simulink model "sampleModel20"  (R2021a)
settings: Solver=VariableStepAuto  StartTime=0.0  StopTime=10.0  RelTol=1e-3
undefined symbols (not defined in the file): DiscIntNeverNeededParam, magnitude, Newton, Raphson
libraries: simulink x274, pid_lib x17
(part 5 of 16)

== system sampleModel20/cfblk84/cfblk10/cfblk11 ==
  cfblk1 : Inport
  cfblk10 : Inport  Port=2
  cfblk11 : Inport  Port=3
  cfblk12 : Inport  Port=4
  cfblk{13..18} (6 alike) : Delay  SampleTime=1
  cfblk3 : Product  Inputs=**
  cfblk4 : Product
  cfblk5 : simulink/Math Operations/MinMax Running Resettable  Function=min  vinit=0.0
  cfblk6 : Reshape
  cfblk7 : Sqrt  Operator=rSqrt  AlgorithmType=Newton-Raphson  SaturateOnIntegerOverflow=on
  cfblk8 : Subsystem
  cfblk9 : Subsystem
  cfblk2 : Outport
  wires:
  cfblk11/1 -> cfblk5/1
  cfblk7/1 -> cfblk4/1
  cfblk3/1 -> cfblk7/1
  cfblk5/1 -> cfblk6/1
  cfblk12/1 -> cfblk9/1(cfblk1)
  cfblk8/2(cfblk7) -> cfblk9/2(cfblk6)
  cfblk1/1 -> cfblk2/1
  cfblk10/1 -> cfblk9/3(cfblk7)
  cfblk4/1 -> cfblk8/2(cfblk5)
  cfblk8/1(cfblk2) -> cfblk13/1
  cfblk13/1 -> cfblk4/2
  cfblk9/1(cfblk2) -> cfblk14/1
  cfblk14/1 -> cfblk3/2
  cfblk9/2(cfblk8) -> cfblk15/1
  cfblk15/1 -> cfblk8/1(cfblk1)
  cfblk9/3(cfblk9) -> cfblk16/1
  cfblk16/1 -> cfblk8/3(cfblk6)
  cfblk8/3(cfblk8) -> cfblk17/1
  cfblk17/1 -> cfblk3/1
  cfblk6/1 -> cfblk18/1
  cfblk18/1 -> cfblk5/2

== system sampleModel20/cfblk84/cfblk10/cfblk9 ==
  cfblk1 : Inport
  cfblk9 : Inport  Port=2
  cfblk10 : Inport  Port=3
  cfblk11 : Delay  SampleTime=1
  cfblk3 : simulink/Math Operations/Slider Gain  gain=1  low=0  high=2
  cfblk4 : Squeeze
  cfblk5 : Math  Operator=log  SaturateOnIntegerOverflow=on
  cfblk6 : PermuteDimensions
  cfblk7 : Trigonometry
  cfblk8 : Subsystem
  cfblk2 : Outport
  wires:
  cfblk9/1 -> cfblk8/1(cfblk1)
  cfblk3/1 -> cfblk6/1
  cfblk1/1 -> cfblk5/1
  cfblk8/1(cfblk2) -> cfblk7/1
  cfblk6/1 -> cfblk4/1
  cfblk5/1 -> cfblk3/1, cfblk8/5(cfblk11), cfblk8/6(cfblk12), cfblk8/7(cfblk13)
  cfblk4/1 -> cfblk8/2(cfblk8)
  cfblk10/1 -> cfblk8/4(cfblk10), cfblk2/1
  cfblk7/1 -> cfblk11/1
  cfblk11/1 -> cfblk8/3(cfblk9)

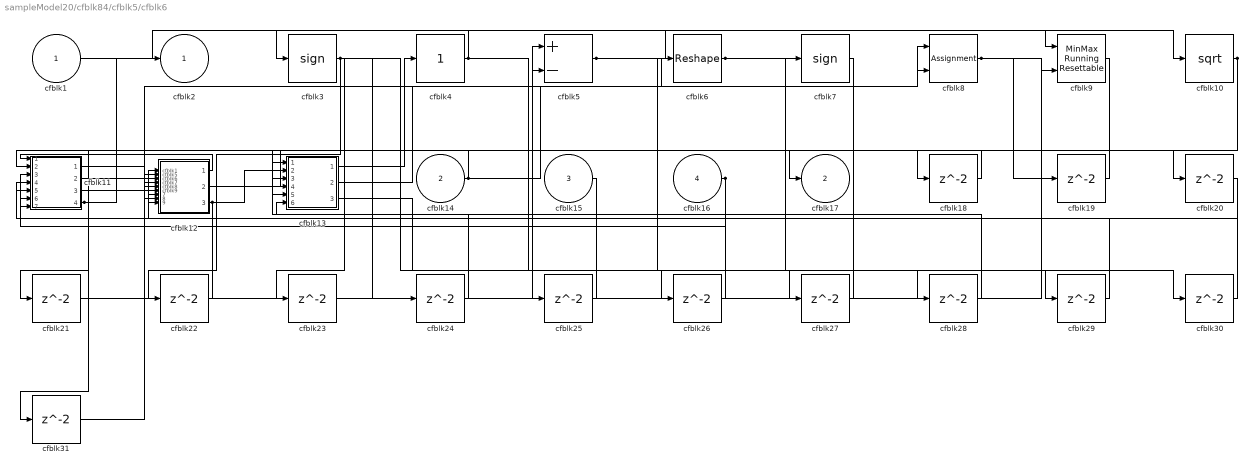
== system sampleModel20/cfblk84/cfblk5/cfblk6 ==
  cfblk1 : Inport
  cfblk14 : Inport  Port=2
  cfblk15 : Inport  Port=3
  cfblk16 : Inport  Port=4
  cfblk10 : Sqrt  SaturateOnIntegerOverflow=on
  cfblk11 : Subsystem
  cfblk12 : Subsystem
  cfblk13 : Subsystem
  cfblk{18..31} (14 alike) : Delay  SampleTime=1
  cfblk3 : Signum
  cfblk4 : simulink/Math Operations/Slider Gain  gain=1  low=0  high=2
  cfblk5 : Sum  Inputs=+-
  cfblk6 : Reshape
  cfblk7 : Signum
  cfblk8 : Assignment  DiagnosticForDimensions=Warning  IndexOptions=Index vector (dialog)  Indices=1  OutputSizes=1
  cfblk9 : simulink/Math Operations/MinMax Running Resettable  Function=min  vinit=0.0
  cfblk2 : Outport
  cfblk17 : Outport  Port=2
  wires:
  cfblk12/1(cfblk2) -> cfblk11/1(cfblk1)
  cfblk8/1 -> cfblk19/1, cfblk20/1
  cfblk15/1 -> cfblk12/1(cfblk1)
  cfblk12/2(cfblk13) -> cfblk17/1
  cfblk14/1 -> cfblk12/2(cfblk5), cfblk8/2
  cfblk16/1 -> cfblk11/3(cfblk7), cfblk12/7(cfblk10)
  cfblk13/1(cfblk2) -> cfblk4/1
  cfblk4/1 -> cfblk3/1, cfblk26/1
  cfblk5/1 -> cfblk10/1, cfblk30/1
  cfblk1/1 -> cfblk9/1
  cfblk13/2(cfblk15) -> cfblk6/1
  cfblk6/1 -> cfblk7/1, cfblk28/1
  cfblk3/1 -> cfblk22/1, cfblk23/1, cfblk24/1, cfblk25/1
  cfblk11/2(cfblk12) -> cfblk8/1
  cfblk10/1 -> cfblk13/5(cfblk13), cfblk21/1
  cfblk9/1 -> cfblk12/5(cfblk8)
  cfblk11/3(cfblk13) -> cfblk5/1
  cfblk11/4(cfblk14) -> cfblk2/1, cfblk31/1
  cfblk12/3(cfblk14) -> cfblk11/6(cfblk10), cfblk13/2(cfblk10), cfblk13/4(cfblk12)
  cfblk11/1(cfblk2) -> cfblk18/1
  cfblk18/1 -> cfblk12/4(cfblk7)
  cfblk19/1 -> cfblk11/2(cfblk6)
  cfblk20/1 -> cfblk11/7(cfblk11)
  cfblk21/1 -> cfblk9/2
  cfblk22/1 -> cfblk11/5(cfblk9)
  cfblk23/1 -> cfblk5/2
  cfblk24/1 -> cfblk13/3(cfblk11)
  cfblk25/1 -> cfblk13/6(cfblk14)
  cfblk26/1 -> cfblk12/9(cfblk12)
  cfblk7/1 -> cfblk27/1
  cfblk27/1 -> cfblk11/4(cfblk8)
  cfblk28/1 -> cfblk13/1(cfblk1)
  cfblk13/3(cfblk16) -> cfblk29/1
  cfblk29/1 -> cfblk12/3(cfblk6)
  cfblk30/1 -> cfblk12/8(cfblk11)
  cfblk31/1 -> cfblk12/6(cfblk9)

== system sampleModel20/cfblk84/cfblk5/cfblk7 ==
  cfblk1 : Inport
  cfblk9 : Inport  Port=2
  cfblk10 : Inport  Port=3
  cfblk{11..15} (5 alike) : Delay  SampleTime=1
  cfblk3 : Product  Inputs=*
  cfblk4 : Signum
  cfblk5 : Subsystem
  cfblk6 : Subsystem
  cfblk7 : Subsystem
  cfblk8 : Subsystem
  cfblk2 : Outport
  wires:
  cfblk9/1 -> cfblk8/1(cfblk1), cfblk8/7(cfblk11), cfblk6/4(cfblk10)
  cfblk4/1 -> cfblk6/1(cfblk1), cfblk5/3(cfblk12), cfblk8/6(cfblk10), cfblk5/6(cfblk15)
  cfblk3/1 -> cfblk6/2(cfblk8), cfblk7/4(cfblk12)
  cfblk1/1 -> cfblk4/1, cfblk7/3(cfblk11)
  cfblk10/1 -> cfblk3/1, cfblk7/5(cfblk13), cfblk5/5(cfblk14)
  cfblk5/1(cfblk2) -> cfblk2/1
  cfblk5/2(cfblk17) -> cfblk8/3(cfblk7), cfblk8/5(cfblk9), cfblk7/6(cfblk14)
  cfblk6/1(cfblk2) -> cfblk5/1(cfblk1), cfblk5/7(cfblk16)
  cfblk8/1(cfblk2) -> cfblk7/1(cfblk1)
  cfblk8/2(cfblk12) -> cfblk7/2(cfblk10), cfblk14/1, cfblk15/1
  cfblk7/1(cfblk2) -> cfblk11/1
  cfblk11/1 -> cfblk8/2(cfblk6)
  cfblk7/2(cfblk15) -> cfblk12/1
  cfblk12/1 -> cfblk6/3(cfblk9)
  cfblk7/3(cfblk16) -> cfblk13/1
  cfblk13/1 -> cfblk8/4(cfblk8)
  cfblk14/1 -> cfblk5/2(cfblk11)
  cfblk15/1 -> cfblk5/4(cfblk13)

== system sampleModel20/cfblk84/cfblk5/cfblk8 ==
  cfblk1 : Inport
  cfblk9 : Inport  Port=2
  cfblk10 : Inport  Port=3
  cfblk11 : Inport  Port=4
  cfblk12 : Inport  Port=5
  cfblk14 : Delay  SampleTime=1
  cfblk15 : Delay  SampleTime=1
  cfblk16 : Delay  SampleTime=1
  cfblk3 : ComplexToRealImag
  cfblk4 : Squeeze
  cfblk5 : simulink/Math Operations/Slider Gain  gain=1  low=0  high=2
  cfblk6 : Assignment  DiagnosticForDimensions=Warning  IndexOptions=Index vector (dialog)  Indices=1  OutputSizes=1
  cfblk7 : Subsystem
  cfblk8 : Subsystem
  cfblk2 : Outport
  cfblk13 : Outport  Port=2
  wires:
  cfblk12/1 -> cfblk13/1
  cfblk9/1 -> cfblk8/1(cfblk1)
  cfblk11/1 -> cfblk8/2(cfblk5), cfblk7/6(cfblk13), cfblk8/5(cfblk8)
  cfblk7/1(cfblk2) -> cfblk5/1
  cfblk5/1 -> cfblk4/1
  cfblk10/1 -> cfblk7/1(cfblk1)
  cfblk8/1(cfblk2) -> cfblk2/1
  cfblk3/1 -> cfblk7/3(cfblk10)
  cfblk8/2(cfblk9) -> cfblk3/1
  cfblk1/1 -> cfblk8/3(cfblk6)
  cfblk7/2(cfblk14) -> cfblk6/1
  cfblk3/2 -> cfblk7/4(cfblk11)
  cfblk7/3(cfblk15) -> cfblk6/2, cfblk16/1
  cfblk4/1 -> cfblk14/1
  cfblk14/1 -> cfblk7/2(cfblk9)
  cfblk6/1 -> cfblk15/1
  cfblk15/1 -> cfblk7/5(cfblk12)
  cfblk16/1 -> cfblk8/4(cfblk7)

== system sampleModel20/cfblk84/cfblk5/cfblk9 ==
  cfblk1 : Inport
  cfblk8 : Inport  Port=2
  cfblk9 : Inport  Port=3
  cfblk12 : Delay  SampleTime=1
  cfblk3 : Polyval  Coefs=[ +2.081618890e-019, -1.441693666e-014, +4.719686976e-010, -8.536869453e-006, +1.621573104e-001, -8.087801117e+001 ]
  cfblk4 : Product
  cfblk5 : UnaryMinus
  cfblk6 : Subsystem
  cfblk7 : Subsystem
  cfblk2 : Outport
  cfblk10 : Outport  Port=2
  cfblk11 : Outport  Port=3
  wires:
  cfblk5/1 -> cfblk10/1, cfblk7/3(cfblk6)
  cfblk3/1 -> cfblk4/1
  cfblk6/1(cfblk2) -> cfblk5/1
  cfblk9/1 -> cfblk4/2
  cfblk1/1 -> cfblk6/1(cfblk1)
  cfblk6/2(cfblk7) -> cfblk2/1
  cfblk8/1 -> cfblk6/3(cfblk6), cfblk7/2(cfblk5), cfblk7/4(cfblk7)
  cfblk7/1(cfblk2) -> cfblk3/1
  cfblk6/3(cfblk8) -> cfblk7/1(cfblk1)
  cfblk7/2(cfblk8) -> cfblk11/1
  cfblk4/1 -> cfblk12/1
  cfblk12/1 -> cfblk6/2(cfblk5)

== system sampleModel20/cfblk84/cfblk6/cfblk4 ==
  cfblk1 : Inport
  cfblk6 : Inport  Port=2
  cfblk7 : Inport  Port=3
  cfblk3 : ComplexToRealImag
  cfblk4 : Gain  Gain=[670276917.632316]
  cfblk5 : Subsystem
  cfblk2 : Outport
  wires:
  cfblk4/1 -> cfblk5/1(cfblk1)
  cfblk3/1 -> cfblk4/1
  cfblk6/1 -> cfblk5/2(cfblk8)
  cfblk1/1 -> cfblk5/3(cfblk9)
  cfblk5/1(cfblk2) -> cfblk2/1
  cfblk7/1 -> cfblk3/1
  cfblk3/2 -> cfblk5/4(cfblk10)

== system sampleModel20/cfblk84/cfblk6/cfblk5 ==
  cfblk1 : Inport
  cfblk11 : Inport  Port=2
  cfblk12 : Inport  Port=3
  cfblk13 : Inport  Port=4
  cfblk10 : Subsystem
  cfblk{14..20} (7 alike) : Delay  SampleTime=1
  cfblk3 : Signum
  cfblk4 : Sqrt  Operator=rSqrt  AlgorithmType=Newton-Raphson  SaturateOnIntegerOverflow=on
  cfblk5 : Signum
  cfblk6 : Subsystem
  cfblk7 : Subsystem
  cfblk8 : Subsystem
  cfblk9 : Subsystem
  cfblk2 : Outport
  wires:
  cfblk5/1 -> cfblk18/1, cfblk19/1, cfblk20/1
  cfblk1/1 -> cfblk4/1, cfblk8/4(cfblk8)
  cfblk10/1(cfblk2) -> cfblk7/1(cfblk1)
  cfblk11/1 -> cfblk10/2(cfblk11)
  cfblk12/1 -> cfblk6/1(cfblk1), cfblk9/4(cfblk12)
  cfblk13/1 -> cfblk3/1, cfblk9/5(cfblk13), cfblk9/6(cfblk14)
  cfblk6/1(cfblk2) -> cfblk9/1(cfblk1)
  cfblk4/1 -> cfblk10/4(cfblk13)
  cfblk10/2(cfblk15) -> cfblk9/2(cfblk10)
  cfblk3/1 -> cfblk2/1, cfblk9/3(cfblk11)
  cfblk8/2(cfblk10) -> cfblk5/1
  cfblk10/3(cfblk16) -> cfblk8/1(cfblk1)
  cfblk7/2(cfblk8) -> cfblk6/2(cfblk10)
  cfblk6/2(cfblk12) -> cfblk8/2(cfblk6), cfblk8/3(cfblk7)
  cfblk7/1(cfblk2) -> cfblk14/1
  cfblk14/1 -> cfblk10/5(cfblk14)
  cfblk9/1(cfblk2) -> cfblk15/1
  cfblk15/1 -> cfblk7/2(cfblk6)
  cfblk9/2(cfblk15) -> cfblk16/1
  cfblk16/1 -> cfblk7/3(cfblk7)
  cfblk8/1(cfblk2) -> cfblk17/1
  cfblk17/1 -> cfblk10/3(cfblk12)
  cfblk18/1 -> cfblk10/1(cfblk1)
  cfblk19/1 -> cfblk6/3(cfblk11)
  cfblk20/1 -> cfblk8/5(cfblk9)

== system sampleModel20/cfblk84/cfblk6/cfblk6 ==
  cfblk1 : Inport
  cfblk7 : Inport  Port=2
  cfblk8 : Inport  Port=3
  cfblk9 : Inport  Port=4
  cfblk10 : Inport  Port=5
  cfblk11 : Inport  Port=6
  cfblk12 : Inport  Port=7
  cfblk13 : Inport  Port=8
  cfblk14 : Inport  Port=9
  cfblk3 : Assignment  DiagnosticForDimensions=Warning  IndexOptions=Index vector (dialog)  Indices=1  OutputSizes=1
  cfblk4 : Product  Inputs=*
  cfblk5 : Subsystem
  cfblk6 : Subsystem
  cfblk2 : Outport
  cfblk15 : Outport  Port=2
  cfblk16 : Outport  Port=3
  wires:
  cfblk13/1 -> cfblk16/1, cfblk5/7(cfblk9)
  cfblk10/1 -> cfblk6/1(cfblk1)
  cfblk6/1(cfblk2) -> cfblk2/1
  cfblk8/1 -> cfblk6/2(cfblk8), cfblk5/8(cfblk10), cfblk5/10(cfblk12)
  cfblk1/1 -> cfblk3/1
  cfblk4/1 -> cfblk15/1
  cfblk5/1(cfblk2) -> cfblk4/1
  cfblk9/1 -> cfblk3/2
  cfblk6/2(cfblk9) -> cfblk5/1(cfblk1)
  cfblk12/1 -> cfblk5/2(cfblk4), cfblk5/9(cfblk11)
  cfblk11/1 -> cfblk5/3(cfblk5)
  cfblk7/1 -> cfblk5/4(cfblk6)
  cfblk14/1 -> cfblk5/5(cfblk7)
  cfblk3/1 -> cfblk5/6(cfblk8)

== system sampleModel20/cfblk84/cfblk7/cfblk10 ==
  cfblk1 : Inport
  cfblk10 : Inport  Port=2
  cfblk11 : Inport  Port=3
  cfblk12 : Inport  Port=4
  cfblk13 : Inport  Port=5
  cfblk14 : Inport  Port=6
  cfblk{18..21} (4 alike) : Delay  SampleTime=1
  cfblk3 : Product
  cfblk4 : ComplexToRealImag
  cfblk5 : ComplexToMagnitudeAngle
  cfblk6 : Subsystem
  cfblk7 : Subsystem
  cfblk8 : Subsystem
  cfblk9 : Subsystem
  cfblk2 : Outport
  cfblk15 : Outport  Port=2
  cfblk16 : Outport  Port=3
  cfblk17 : Outport  Port=4
  wires:
  cfblk4/1 -> cfblk9/1(cfblk1)
  cfblk8/1(cfblk2) -> cfblk16/1
  cfblk7/1(cfblk2) -> cfblk17/1
  cfblk10/1 -> cfblk7/1(cfblk1)
  cfblk6/1(cfblk2) -> cfblk4/1
  cfblk3/1 -> cfblk6/2(cfblk6), cfblk19/1, cfblk21/1
  cfblk9/1(cfblk2) -> cfblk7/2(cfblk7)
  cfblk5/1 -> cfblk15/1
  cfblk14/1 -> cfblk3/1
  cfblk5/2 -> cfblk3/2, cfblk6/3(cfblk7)
  cfblk4/2 -> cfblk7/3(cfblk8), cfblk20/1
  cfblk6/2(cfblk9) -> cfblk9/2(cfblk5)
  cfblk1/1 -> cfblk8/2(cfblk8), cfblk8/5(cfblk11)
  cfblk13/1 -> cfblk9/3(cfblk6)
  cfblk7/2(cfblk10) -> cfblk2/1, cfblk18/1
  cfblk8/2(cfblk14) -> cfblk7/4(cfblk9)
  cfblk6/3(cfblk10) -> cfblk9/4(cfblk7)
  cfblk12/1 -> cfblk8/3(cfblk9), cfblk9/6(cfblk9)
  cfblk8/3(cfblk15) -> cfblk5/1
  cfblk8/4(cfblk16) -> cfblk9/5(cfblk8)
  cfblk11/1 -> cfblk6/1(cfblk1), cfblk6/4(cfblk8)
  cfblk18/1 -> cfblk8/7(cfblk13)
  cfblk19/1 -> cfblk8/1(cfblk1)
  cfblk20/1 -> cfblk8/4(cfblk10)
  cfblk21/1 -> cfblk8/6(cfblk12)

== system sampleModel20/cfblk84/cfblk7/cfblk9 ==
  cfblk1 : Inport
  cfblk8 : Inport  Port=2
  cfblk9 : Inport  Port=3
  cfblk10 : Inport  Port=4
  cfblk11 : Inport  Port=5
  cfblk12 : Inport  Port=6
  cfblk15 : Delay  SampleTime=1
  cfblk3 : Sum  Inputs=|++
  cfblk4 : Product  Inputs=**
  cfblk5 : Sum  Inputs=+
  cfblk6 : Sum  Inputs=+
  cfblk7 : Subsystem
  cfblk2 : Outport
  cfblk13 : Outport  Port=2
  cfblk14 : Outport  Port=3
  wires:
  cfblk11/1 -> cfblk14/1
  cfblk7/1(cfblk2) -> cfblk5/1
  cfblk3/1 -> cfblk13/1
  cfblk9/1 -> cfblk7/1(cfblk1)
  cfblk4/1 -> cfblk3/1
  cfblk6/1 -> cfblk3/2
  cfblk12/1 -> cfblk6/1
  cfblk5/1 -> cfblk4/1, cfblk15/1
  cfblk8/1 -> cfblk7/2(cfblk12)
  cfblk7/2(cfblk16) -> cfblk2/1
  cfblk1/1 -> cfblk7/3(cfblk13)
  cfblk10/1 -> cfblk7/4(cfblk14)
  cfblk7/3(cfblk17) -> cfblk4/2
  cfblk15/1 -> cfblk7/5(cfblk15)

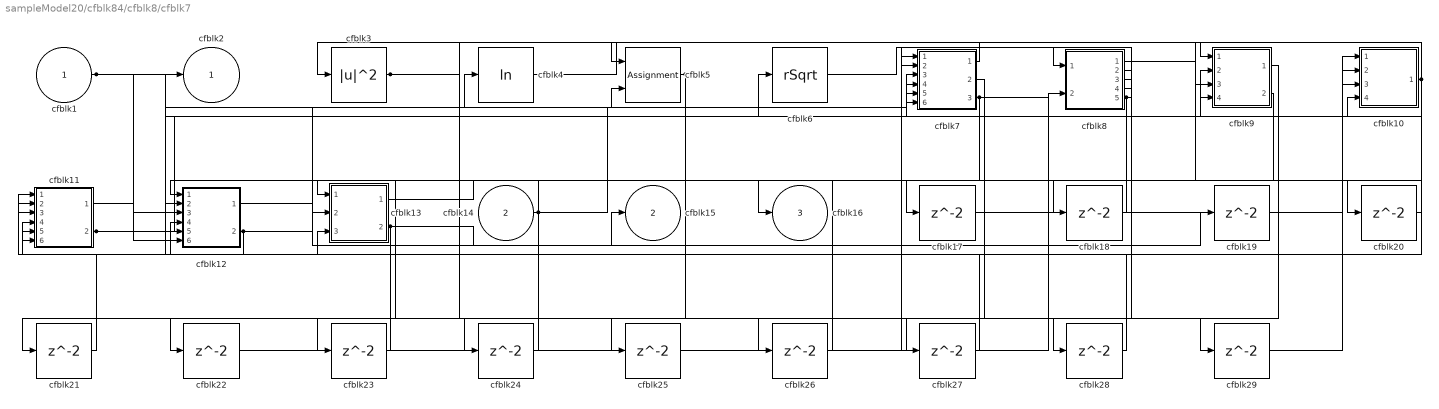
== system sampleModel20/cfblk84/cfblk8/cfblk7 ==
  cfblk1 : Inport
  cfblk14 : Inport  Port=2
  cfblk10 : Subsystem
  cfblk11 : Subsystem
  cfblk12 : Subsystem
  cfblk13 : Subsystem
  cfblk{17..29} (13 alike) : Delay  SampleTime=1
  cfblk3 : Math  Operator=magnitude^2  SaturateOnIntegerOverflow=on
  cfblk4 : Math  Operator=log  SaturateOnIntegerOverflow=on
  cfblk5 : Assignment  DiagnosticForDimensions=Warning  IndexOptions=Index vector (dialog)  Indices=1  OutputSizes=1
  cfblk6 : Sqrt  Operator=rSqrt  AlgorithmType=Newton-Raphson  SaturateOnIntegerOverflow=on
  cfblk7 : Subsystem
  cfblk8 : Subsystem
  cfblk9 : Subsystem
  cfblk2 : Outport
  cfblk15 : Outport  Port=2
  cfblk16 : Outport  Port=3
  wires:
  cfblk4/1 -> cfblk9/1(cfblk1)
  cfblk5/1 -> cfblk4/1, cfblk24/1
  cfblk3/1 -> cfblk9/3(cfblk9), cfblk29/1
  cfblk11/1(cfblk2) -> cfblk2/1
  cfblk6/1 -> cfblk8/1(cfblk1)
  cfblk11/2(cfblk15) -> cfblk6/1, cfblk5/2
  cfblk10/1(cfblk2) -> cfblk13/3(cfblk9), cfblk3/1, cfblk7/6(cfblk13)
  cfblk12/2(cfblk12) -> cfblk11/5(cfblk13), cfblk7/5(cfblk12), cfblk19/1
  cfblk1/1 -> cfblk10/4(cfblk9), cfblk12/3(cfblk8), cfblk12/6(cfblk11)
  cfblk13/2(cfblk10) -> cfblk15/1, cfblk12/4(cfblk9)
  cfblk14/1 -> cfblk12/1(cfblk1), cfblk7/4(cfblk11), cfblk11/4(cfblk12)
  cfblk8/3(cfblk14) -> cfblk7/2(cfblk9)
  cfblk7/1(cfblk2) -> cfblk5/1
  cfblk8/4(cfblk15) -> cfblk7/3(cfblk10)
  cfblk7/3(cfblk15) -> cfblk9/2(cfblk8), cfblk9/4(cfblk10), cfblk16/1
  cfblk8/5(cfblk16) -> cfblk26/1, cfblk27/1, cfblk28/1
  cfblk13/1(cfblk2) -> cfblk17/1
  cfblk17/1 -> cfblk10/2(cfblk7)
  cfblk12/1(cfblk2) -> cfblk18/1
  cfblk18/1 -> cfblk13/2(cfblk8)
  cfblk19/1 -> cfblk10/3(cfblk8)
  cfblk8/1(cfblk2) -> cfblk20/1
  cfblk20/1 -> cfblk13/1(cfblk1)
  cfblk8/2(cfblk13) -> cfblk21/1
  cfblk21/1 -> cfblk11/2(cfblk10)
  cfblk9/1(cfblk2) -> cfblk22/1
  cfblk22/1 -> cfblk7/1(cfblk1)
  cfblk9/2(cfblk11) -> cfblk23/1
  cfblk23/1 -> cfblk11/1(cfblk1)
  cfblk24/1 -> cfblk12/5(cfblk10)
  cfblk7/2(cfblk14) -> cfblk25/1
  cfblk25/1 -> cfblk8/2(cfblk12)
  cfblk26/1 -> cfblk11/3(cfblk11)
  cfblk27/1 -> cfblk11/6(cfblk14)
  cfblk28/1 -> cfblk12/2(cfblk7)
  cfblk29/1 -> cfblk10/1(cfblk1)

== system sampleModel20/cfblk84/cfblk8/cfblk8 ==
  cfblk1 : Inport
  cfblk11 : Inport  Port=2
  cfblk10 : Subsystem
  cfblk{12..16} (5 alike) : Delay  SampleTime=1
  cfblk3 : Sqrt  SaturateOnIntegerOverflow=on
  cfblk4 : Sqrt  SaturateOnIntegerOverflow=on
  cfblk5 : Signum
  cfblk6 : Polyval  Coefs=[ +2.081618890e-019, -1.441693666e-014, +4.719686976e-010, -8.536869453e-006, +1.621573104e-001, -8.087801117e+001 ]
  cfblk7 : Subsystem
  cfblk8 : Subsystem
  cfblk9 : Subsystem
  cfblk2 : Outport
  wires:
  cfblk9/1(cfblk2) -> cfblk3/1, cfblk15/1
  cfblk8/1(cfblk2) -> cfblk4/1
  cfblk1/1 -> cfblk6/1, cfblk8/2(cfblk3), cfblk7/4(cfblk12)
  cfblk6/1 -> cfblk10/2(cfblk7), cfblk2/1, cfblk8/3(cfblk4)
  cfblk7/3(cfblk16) -> cfblk5/1
  cfblk4/1 -> cfblk7/6(cfblk14), cfblk16/1
  cfblk11/1 -> cfblk9/2(cfblk7), cfblk8/4(cfblk5)
  cfblk3/1 -> cfblk7/2(cfblk10)
  cfblk8/2(cfblk6) -> cfblk10/3(cfblk8)
  cfblk10/1(cfblk2) -> cfblk9/3(cfblk8), cfblk7/3(cfblk11), cfblk7/5(cfblk13)
  cfblk8/3(cfblk7) -> cfblk10/4(cfblk9)
  cfblk7/1(cfblk2) -> cfblk12/1
  cfblk12/1 -> cfblk9/1(cfblk1)
  cfblk7/2(cfblk15) -> cfblk13/1
  cfblk13/1 -> cfblk10/1(cfblk1)
  cfblk5/1 -> cfblk14/1
  cfblk14/1 -> cfblk7/1(cfblk1)
  cfblk15/1 -> cfblk10/5(cfblk10)
  cfblk16/1 -> cfblk8/1(cfblk1)

== system sampleModel20/cfblk84/cfblk8/cfblk9 ==
  cfblk1 : Inport
  cfblk7 : Inport  Port=2
  cfblk8 : Inport  Port=3
  cfblk9 : Inport  Port=4
  cfblk11 : Delay  SampleTime=1
  cfblk12 : Delay  SampleTime=1
  cfblk13 : Delay  SampleTime=1
  cfblk3 : DiscreteStateSpace
  cfblk4 : Subsystem
  cfblk5 : Subsystem
  cfblk6 : Subsystem
  cfblk2 : Outport
  cfblk10 : Outport  Port=2
  wires:
  cfblk5/2(cfblk10) -> cfblk2/1
  cfblk5/3(cfblk11) -> cfblk3/1, cfblk6/7(cfblk16)
  cfblk7/1 -> cfblk5/1(cfblk1), cfblk6/5(cfblk14), cfblk6/6(cfblk15)
  cfblk4/1(cfblk2) -> cfblk5/2(cfblk7)
  cfblk8/1 -> cfblk5/3(cfblk8), cfblk6/2(cfblk11), cfblk6/3(cfblk12)
  cfblk3/1 -> cfblk10/1, cfblk6/1(cfblk1), cfblk6/4(cfblk13)
  cfblk9/1 -> cfblk5/4(cfblk9)
  cfblk1/1 -> cfblk4/2(cfblk5)
  cfblk5/1(cfblk2) -> cfblk11/1
  cfblk11/1 -> cfblk4/1(cfblk1)
  cfblk6/1(cfblk2) -> cfblk12/1
  cfblk12/1 -> cfblk4/3(cfblk6)
  cfblk6/2(cfblk17) -> cfblk13/1
  cfblk13/1 -> cfblk4/4(cfblk7)

== system sampleModel20/cfblk84/cfblk9/cfblk5 ==
  cfblk1 : Inport
  cfblk9 : Inport  Port=2
  cfblk10 : Inport  Port=3
  cfblk11 : Inport  Port=4
  cfblk12 : Delay  SampleTime=1
  cfblk13 : Delay  SampleTime=1
  cfblk3 : DotProduct  InputSameDT=on  OutDataTypeStr=Inherit: Inherit via internal rule
  cfblk4 : Math  Operator=log10  SaturateOnIntegerOverflow=on
  cfblk5 : simulink/Math Operations/MinMax Running Resettable  Function=min  vinit=0.0
  cfblk6 : simulink/Math Operations/Slider Gain  gain=1  low=0  high=2
  cfblk7 : Assignment  DiagnosticForDimensions=Warning  IndexOptions=Index vector (dialog)  Indices=1  OutputSizes=1
  cfblk8 : Subsystem
  cfblk2 : Outport
  wires:
  cfblk11/1 -> cfblk2/1
  cfblk5/1 -> cfblk8/1(cfblk1)
  cfblk1/1 -> cfblk7/1
  cfblk10/1 -> cfblk7/2
  cfblk3/1 -> cfblk5/1
  cfblk9/1 -> cfblk3/1
  cfblk4/1 -> cfblk6/1
  cfblk8/1(cfblk2) -> cfblk4/1
  cfblk6/1 -> cfblk12/1
  cfblk12/1 -> cfblk5/2
  cfblk8/2(cfblk8) -> cfblk13/1
  cfblk13/1 -> cfblk3/2

== system sampleModel20/cfblk84/cfblk9/cfblk6 ==
  cfblk1 : Inport
  cfblk9 : Inport  Port=2
  cfblk10 : Inport  Port=3
  cfblk11 : Inport  Port=4
  cfblk12 : Inport  Port=5
  cfblk13 : Inport  Port=6
  cfblk14 : Inport  Port=7
  cfblk15 : Inport  Port=8
  cfblk{17..21} (5 alike) : Delay  SampleTime=1
  cfblk3 : ComplexToRealImag
  cfblk4 : Subsystem
  cfblk5 : Subsystem
  cfblk6 : Subsystem
  cfblk7 : Subsystem
  cfblk8 : Subsystem
  cfblk2 : Outport
  cfblk16 : Outport  Port=2
  wires:
  cfblk8/1(cfblk2) -> cfblk16/1
  cfblk14/1 -> cfblk8/1(cfblk1), cfblk5/2(cfblk6)
  cfblk1/1 -> cfblk2/1, cfblk6/6(cfblk11)
  cfblk15/1 -> cfblk7/1(cfblk1)
  cfblk11/1 -> cfblk7/2(cfblk9), cfblk5/3(cfblk7), cfblk6/4(cfblk9)
  cfblk6/1(cfblk2) -> cfblk7/3(cfblk10), cfblk5/4(cfblk8)
  cfblk12/1 -> cfblk6/2(cfblk7), cfblk4/8(cfblk12)
  cfblk10/1 -> cfblk8/2(cfblk14), cfblk4/5(cfblk9)
  cfblk13/1 -> cfblk4/1(cfblk1), cfblk4/7(cfblk11)
  cfblk7/1(cfblk2) -> cfblk3/1
  cfblk3/2 -> cfblk4/2(cfblk6)
  cfblk8/2(cfblk15) -> cfblk7/5(cfblk12)
  cfblk9/1 -> cfblk4/3(cfblk7), cfblk6/3(cfblk8), cfblk5/5(cfblk9)
  cfblk4/2(cfblk14) -> cfblk19/1, cfblk20/1
  cfblk8/3(cfblk16) -> cfblk7/7(cfblk14), cfblk7/9(cfblk16)
  cfblk7/2(cfblk17) -> cfblk5/1(cfblk1), cfblk21/1
  cfblk5/1(cfblk2) -> cfblk4/4(cfblk8), cfblk4/6(cfblk10), cfblk4/9(cfblk13)
  cfblk3/1 -> cfblk17/1
  cfblk17/1 -> cfblk6/1(cfblk1)
  cfblk4/1(cfblk2) -> cfblk18/1
  cfblk18/1 -> cfblk7/4(cfblk11)
  cfblk19/1 -> cfblk7/6(cfblk13)
  cfblk20/1 -> cfblk7/8(cfblk15)
  cfblk21/1 -> cfblk6/5(cfblk10)

== system sampleModel20/cfblk84/cfblk9/cfblk7 ==
  cfblk1 : Inport
  cfblk9 : Inport  Port=2
  cfblk10 : Inport  Port=3
  cfblk11 : Inport  Port=4
  cfblk12 : Inport  Port=5
  cfblk{13..18} (6 alike) : Delay  SampleTime=1
  cfblk3 : Abs
  cfblk4 : simulink/Math Operations/MinMax Running Resettable  Function=min  vinit=0.0
  cfblk5 : Subsystem
  cfblk6 : Subsystem
  cfblk7 : Subsystem
  cfblk8 : Subsystem
  cfblk2 : Outport
  wires:
  cfblk10/1 -> cfblk6/1(cfblk1)
  cfblk8/1(cfblk2) -> cfblk5/1(cfblk1)
  cfblk11/1 -> cfblk2/1
  cfblk8/2(cfblk7) -> cfblk3/1
  cfblk12/1 -> cfblk7/1(cfblk1)
  cfblk1/1 -> cfblk7/3(cfblk7)
  cfblk9/1 -> cfblk5/2(cfblk5)
  cfblk7/1(cfblk2) -> cfblk8/2(cfblk6)
  cfblk5/3(cfblk8) -> cfblk6/2(cfblk6)
  cfblk5/4(cfblk9) -> cfblk6/3(cfblk7)
  cfblk7/2(cfblk11) -> cfblk4/1
  cfblk5/5(cfblk10) -> cfblk4/2
  cfblk5/1(cfblk2) -> cfblk13/1
  cfblk13/1 -> cfblk7/5(cfblk9)
  cfblk5/2(cfblk7) -> cfblk14/1
  cfblk14/1 -> cfblk7/6(cfblk10)
  cfblk6/1(cfblk2) -> cfblk15/1
  cfblk15/1 -> cfblk7/4(cfblk8)
  cfblk6/2(cfblk8) -> cfblk16/1
  cfblk16/1 -> cfblk5/3(cfblk6)
  cfblk4/1 -> cfblk17/1
  cfblk17/1 -> cfblk7/2(cfblk6)
  cfblk3/1 -> cfblk18/1
  cfblk18/1 -> cfblk8/1(cfblk1)

== system sampleModel20/cfblk85/cfblk10/cfblk6 ==
  cfblk1 : Inport
  cfblk7 : Inport  Port=2
  cfblk8 : Inport  Port=3
  cfblk9 : Inport  Port=4
  cfblk10 : Inport  Port=5
  cfblk11 : Inport  Port=6
  cfblk12 : Inport  Port=7
  cfblk14 : Delay  SampleTime=1
  cfblk3 : Subsystem
  cfblk4 : Subsystem
  cfblk5 : Subsystem
  cfblk6 : Subsystem
  cfblk2 : Outport
  cfblk13 : Outport  Port=2
  wires:
  cfblk7/1 -> cfblk6/1(cfblk1)
  cfblk12/1 -> cfblk4/1(cfblk1), cfblk3/7(cfblk15)
  cfblk10/1 -> cfblk13/1, cfblk3/4(cfblk12), cfblk3/5(cfblk13)
  cfblk11/1 -> cfblk5/1(cfblk1)
  cfblk1/1 -> cfblk4/2(cfblk11), cfblk3/3(cfblk11)
  cfblk9/1 -> cfblk4/3(cfblk12)
  cfblk8/1 -> cfblk6/2(cfblk5), cfblk3/6(cfblk14)
  cfblk6/1(cfblk2) -> cfblk5/2(cfblk10)
  cfblk3/1(cfblk2) -> cfblk6/3(cfblk6)
  cfblk3/2(cfblk16) -> cfblk6/4(cfblk7)
  cfblk4/1(cfblk2) -> cfblk2/1
  cfblk4/2(cfblk14) -> cfblk3/1(cfblk1), cfblk3/2(cfblk10)
  cfblk3/3(cfblk17) -> cfblk6/5(cfblk8)
  cfblk5/1(cfblk2) -> cfblk14/1
  cfblk14/1 -> cfblk4/4(cfblk13)

== system sampleModel20/cfblk85/cfblk9/cfblk6 ==
  cfblk1 : Inport
  cfblk6 : Inport  Port=2
  cfblk7 : Inport  Port=3
  cfblk8 : Inport  Port=4
  cfblk9 : Inport  Port=5
  cfblk3 : Gain  Gain=[-520885476.309207]
  cfblk4 : Trigonometry
  cfblk5 : Subsystem
  cfblk2 : Outport
  cfblk10 : Outport  Port=2
  wires:
  cfblk7/1 -> cfblk10/1, cfblk5/4(cfblk9)
  cfblk3/1 -> cfblk2/1
  cfblk8/1 -> cfblk5/1(cfblk1)
  cfblk6/1 -> cfblk4/1
  cfblk4/1 -> cfblk5/2(cfblk7)
  cfblk1/1 -> cfblk3/1
  cfblk9/1 -> cfblk5/3(cfblk8), cfblk5/5(cfblk10)

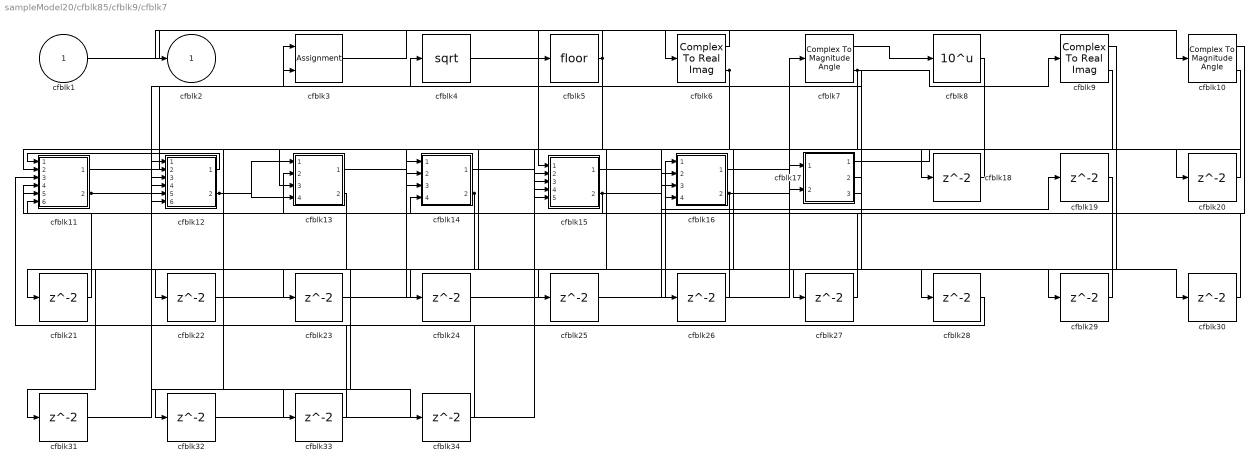
== system sampleModel20/cfblk85/cfblk9/cfblk7 ==
  cfblk1 : Inport
  cfblk10 : ComplexToMagnitudeAngle
  cfblk11 : Subsystem
  cfblk12 : Subsystem
  cfblk13 : Subsystem
  cfblk14 : Subsystem
  cfblk15 : Subsystem
  cfblk16 : Subsystem
  cfblk17 : Subsystem
  cfblk{18..34} (17 alike) : Delay  SampleTime=1
  cfblk3 : Assignment  DiagnosticForDimensions=Warning  IndexOptions=Index vector (dialog)  Indices=1  OutputSizes=1
  cfblk4 : Sqrt  SaturateOnIntegerOverflow=on
  cfblk5 : Rounding
  cfblk6 : ComplexToRealImag
  cfblk7 : ComplexToMagnitudeAngle
  cfblk8 : Math  Operator=10^u  SaturateOnIntegerOverflow=on
  cfblk9 : ComplexToRealImag
  cfblk2 : Outport
  wires:
  cfblk7/1 -> cfblk8/1
  cfblk7/2 -> cfblk9/1, cfblk25/1, cfblk26/1, cfblk27/1
  cfblk1/1 -> cfblk6/1
  cfblk11/1(cfblk2) -> cfblk4/1
  cfblk5/1 -> cfblk2/1, cfblk12/4(cfblk8)
  cfblk12/1(cfblk2) -> cfblk11/1(cfblk1)
  cfblk4/1 -> cfblk15/1(cfblk1)
  cfblk16/1(cfblk2) -> cfblk7/1
  cfblk11/2(cfblk13) -> cfblk3/1, cfblk34/1
  cfblk12/2(cfblk11) -> cfblk13/1(cfblk1), cfblk13/4(cfblk9)
  cfblk3/1 -> cfblk10/1
  cfblk14/1(cfblk2) -> cfblk17/2(cfblk7)
  cfblk10/1 -> cfblk16/1(cfblk1)
  cfblk14/2(cfblk13) -> cfblk32/1, cfblk33/1
  cfblk16/2(cfblk9) -> cfblk13/2(cfblk7), cfblk28/1, cfblk29/1
  cfblk10/2 -> cfblk16/3(cfblk7)
  cfblk6/1 -> cfblk5/1
  cfblk6/2 -> cfblk14/3(cfblk11), cfblk15/5(cfblk14), cfblk13/3(cfblk8), cfblk12/6(cfblk10)
  cfblk17/3(cfblk9) -> cfblk3/2
  cfblk15/2(cfblk15) -> cfblk14/4(cfblk12), cfblk19/1
  cfblk15/1(cfblk2) -> cfblk18/1
  cfblk18/1 -> cfblk12/2(cfblk6)
  cfblk19/1 -> cfblk11/5(cfblk11)
  cfblk17/1(cfblk2) -> cfblk20/1
  cfblk20/1 -> cfblk11/2(cfblk8)
  cfblk17/2(cfblk8) -> cfblk21/1
  cfblk21/1 -> cfblk11/4(cfblk10)
  cfblk8/1 -> cfblk22/1
  cfblk22/1 -> cfblk14/1(cfblk1)
  cfblk9/1 -> cfblk23/1
  cfblk23/1 -> cfblk17/1(cfblk1)
  cfblk9/2 -> cfblk24/1
  cfblk24/1 -> cfblk16/2(cfblk6)
  cfblk25/1 -> cfblk16/4(cfblk8)
  cfblk26/1 -> cfblk11/6(cfblk12)
  cfblk27/1 -> cfblk15/4(cfblk13)
  cfblk28/1 -> cfblk11/3(cfblk9)
  cfblk29/1 -> cfblk15/3(cfblk12)
  cfblk13/1(cfblk2) -> cfblk30/1
  cfblk30/1 -> cfblk14/2(cfblk10)
  cfblk13/2(cfblk10) -> cfblk31/1
  cfblk31/1 -> cfblk12/1(cfblk1)
  cfblk32/1 -> cfblk15/2(cfblk11)
  cfblk33/1 -> cfblk12/5(cfblk9)
  cfblk34/1 -> cfblk12/3(cfblk7)

== system sampleModel20/cfblk85/cfblk9/cfblk8 ==
  cfblk1 : Inport
  cfblk10 : Inport  Port=2
  cfblk11 : Inport  Port=3
  cfblk12 : Inport  Port=4
  cfblk13 : Inport  Port=5
  cfblk{14..20} (7 alike) : Delay  SampleTime=1
  cfblk3 : DotProduct  InputSameDT=on  OutDataTypeStr=Inherit: Inherit via internal rule
  cfblk4 : Signum
  cfblk5 : Sin  TimeSource=Use external signal  SampleTime=0
  cfblk6 : Gain  Gain=[985385243.244329]
  cfblk7 : Subsystem
  cfblk8 : Subsystem
  cfblk9 : Subsystem
  cfblk2 : Outport
  wires:
  cfblk8/1(cfblk2) -> cfblk5/1
  cfblk7/1(cfblk2) -> cfblk4/1
  cfblk6/1 -> cfblk15/1, cfblk16/1, cfblk17/1
  cfblk12/1 -> cfblk7/2(cfblk8), cfblk9/4(cfblk8)
  cfblk13/1 -> cfblk2/1, cfblk8/5(cfblk7), cfblk8/6(cfblk8)
  cfblk10/1 -> cfblk9/1(cfblk1)
  cfblk11/1 -> cfblk3/1, cfblk8/7(cfblk9)
  cfblk1/1 -> cfblk8/2(cfblk4)
  cfblk9/1(cfblk2) -> cfblk7/3(cfblk9)
  cfblk7/2(cfblk14) -> cfblk6/1
  cfblk3/1 -> cfblk9/2(cfblk6), cfblk7/7(cfblk13)
  cfblk5/1 -> cfblk3/2, cfblk20/1
  cfblk9/2(cfblk10) -> cfblk7/4(cfblk10)
  cfblk9/3(cfblk11) -> cfblk7/5(cfblk11)
  cfblk4/1 -> cfblk14/1
  cfblk14/1 -> cfblk8/1(cfblk1)
  cfblk15/1 -> cfblk7/1(cfblk1)
  cfblk16/1 -> cfblk7/6(cfblk12)
  cfblk17/1 -> cfblk9/5(cfblk9)
  cfblk7/3(cfblk15) -> cfblk18/1
  cfblk18/1 -> cfblk9/3(cfblk7)
  cfblk7/4(cfblk16) -> cfblk19/1
  cfblk19/1 -> cfblk8/3(cfblk5)
  cfblk20/1 -> cfblk8/4(cfblk6)

== system sampleModel20/cfblk85/cfblk9/cfblk9 ==
  cfblk1 : Inport
  cfblk11 : Inport  Port=2
  cfblk12 : Inport  Port=3
  cfblk10 : Subsystem
  cfblk14 : Delay  SampleTime=1
  cfblk15 : Delay  SampleTime=1
  cfblk3 : Rounding
  cfblk4 : Abs
  cfblk5 : ComplexToMagnitudeAngle
  cfblk6 : Sum  Inputs=+
  cfblk7 : Subsystem
  cfblk8 : Subsystem
  cfblk9 : Subsystem
  cfblk2 : Outport
  cfblk13 : Outport  Port=2
  wires:
  cfblk3/1 -> cfblk6/1
  cfblk1/1 -> cfblk3/1, cfblk7/3(cfblk12), cfblk8/5(cfblk11)
  cfblk10/1(cfblk2) -> cfblk2/1
  cfblk6/1 -> cfblk9/1(cfblk1), cfblk8/4(cfblk10)
  cfblk8/1(cfblk2) -> cfblk7/1(cfblk1)
  cfblk12/1 -> cfblk5/1, cfblk10/2(cfblk8), cfblk7/8(cfblk17)
  cfblk11/1 -> cfblk13/1, cfblk7/5(cfblk14)
  cfblk5/1 -> cfblk4/1
  cfblk7/1(cfblk2) -> cfblk14/1, cfblk15/1
  cfblk8/2(cfblk13) -> cfblk7/2(cfblk11)
  cfblk9/1(cfblk2) -> cfblk8/2(cfblk8), cfblk7/4(cfblk13), cfblk10/3(cfblk9)
  cfblk4/1 -> cfblk9/2(cfblk7), cfblk10/1(cfblk1), cfblk7/6(cfblk15)
  cfblk5/2 -> cfblk9/3(cfblk8)
  cfblk10/2(cfblk10) -> cfblk8/3(cfblk9), cfblk7/7(cfblk16)
  cfblk14/1 -> cfblk8/1(cfblk1)
  cfblk15/1 -> cfblk8/6(cfblk12)

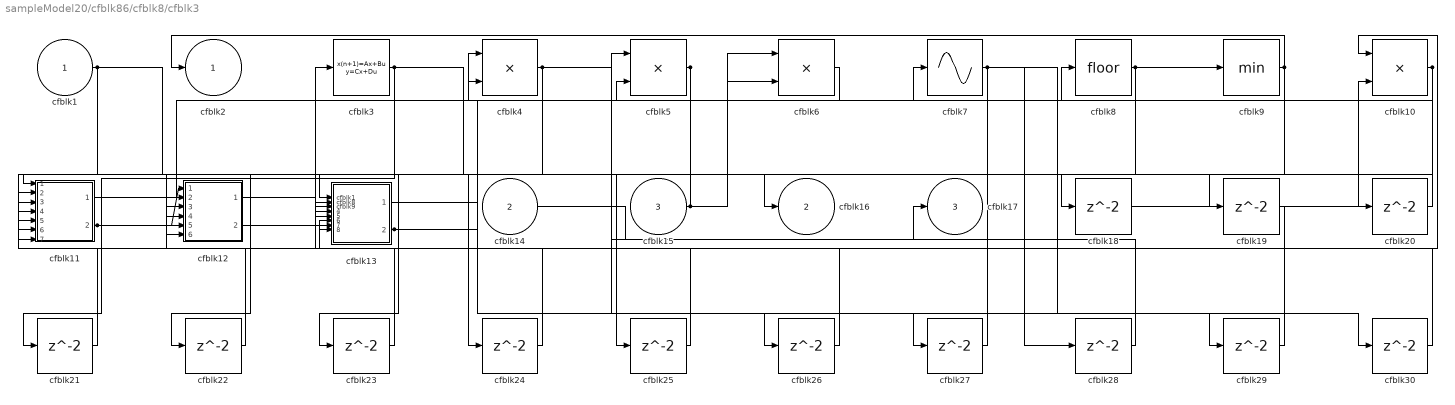
== system sampleModel20/cfblk86/cfblk8/cfblk3 ==
  cfblk1 : Inport
  cfblk14 : Inport  Port=2
  cfblk15 : Inport  Port=3
  cfblk10 : Product
  cfblk11 : Subsystem
  cfblk12 : Subsystem
  cfblk13 : Subsystem
  cfblk{18..30} (13 alike) : Delay  SampleTime=1
  cfblk3 : DiscreteStateSpace
  cfblk4 : Product
  cfblk5 : Product  Inputs=**
  cfblk6 : Product  Inputs=**
  cfblk7 : Sin  TimeSource=Use external signal  SampleTime=0
  cfblk8 : Rounding
  cfblk9 : MinMax
  cfblk2 : Outport
  cfblk16 : Outport  Port=2
  cfblk17 : Outport  Port=3
  wires:
  cfblk9/1 -> cfblk2/1, cfblk22/1, cfblk23/1, cfblk24/1
  cfblk6/1 -> cfblk4/1
  cfblk1/1 -> cfblk16/1, cfblk11/7(cfblk15)
  cfblk14/1 -> cfblk17/1
  cfblk10/1 -> cfblk4/2, cfblk27/1
  cfblk13/1(cfblk2) -> cfblk10/1
  cfblk15/1 -> cfblk11/1(cfblk1), cfblk12/3(cfblk13), cfblk6/1, cfblk6/2
  cfblk13/2(cfblk15) -> cfblk7/1, cfblk30/1
  cfblk7/1 -> cfblk12/2(cfblk12), cfblk28/1, cfblk29/1
  cfblk4/1 -> cfblk12/5(cfblk15), cfblk12/6(cfblk16), cfblk18/1, cfblk19/1, cfblk26/1
  cfblk8/1 -> cfblk9/1, cfblk25/1
  cfblk11/1(cfblk2) -> cfblk5/2
  cfblk5/1 -> cfblk13/1(cfblk1), cfblk13/4(cfblk10)
  cfblk12/1(cfblk2) -> cfblk3/1
  cfblk12/2(cfblk17) -> cfblk8/1
  cfblk11/2(cfblk16) -> cfblk12/1(cfblk1), cfblk13/6(cfblk12)
  cfblk3/1 -> cfblk20/1, cfblk21/1
  cfblk18/1 -> cfblk10/2
  cfblk19/1 -> cfblk11/5(cfblk13)
  cfblk20/1 -> cfblk13/2(cfblk8)
  cfblk21/1 -> cfblk11/3(cfblk11)
  cfblk22/1 -> cfblk12/4(cfblk14)
  cfblk23/1 -> cfblk13/5(cfblk11)
  cfblk24/1 -> cfblk13/7(cfblk13)
  cfblk25/1 -> cfblk11/4(cfblk12)
  cfblk26/1 -> cfblk13/8(cfblk14)
  cfblk27/1 -> cfblk13/3(cfblk9)
  cfblk28/1 -> cfblk5/1
  cfblk29/1 -> cfblk11/6(cfblk14)
  cfblk30/1 -> cfblk11/2(cfblk10)

== system sampleModel20/cfblk86/cfblk9/cfblk10 ==
  cfblk1 : Inport
  cfblk8 : Inport  Port=2
  cfblk{10..17} (8 alike) : Delay  SampleTime=1
  cfblk3 : Sum  Inputs=+-
  cfblk4 : Bias  Bias=[181588559.530365]
  cfblk5 : Subsystem
  cfblk6 : Subsystem
  cfblk7 : Subsystem
  cfblk2 : Outport
  cfblk9 : Outport  Port=2
  wires:
  cfblk3/1 -> cfblk9/1, cfblk11/1, cfblk12/1, cfblk13/1, cfblk14/1
  cfblk6/1(cfblk2) -> cfblk5/1(cfblk1)
  cfblk7/1(cfblk2) -> cfblk4/1
  cfblk4/1 -> cfblk6/5(cfblk9), cfblk10/1
  cfblk5/1(cfblk2) -> cfblk3/1
  cfblk7/2(cfblk9) -> cfblk2/1
  cfblk1/1 -> cfblk7/2(cfblk4), cfblk7/6(cfblk8)
  cfblk8/1 -> cfblk3/2, cfblk5/3(cfblk11), cfblk6/4(cfblk8), cfblk6/6(cfblk10), cfblk6/7(cfblk11)
  cfblk7/3(cfblk10) -> cfblk5/2(cfblk10)
  cfblk5/2(cfblk12) -> cfblk15/1, cfblk16/1, cfblk17/1
  cfblk10/1 -> cfblk7/1(cfblk1)
  cfblk11/1 -> cfblk6/1(cfblk1)
  cfblk12/1 -> cfblk7/4(cfblk6)
  cfblk13/1 -> cfblk6/2(cfblk6)
  cfblk14/1 -> cfblk6/8(cfblk12)
  cfblk15/1 -> cfblk7/3(cfblk5)
  cfblk16/1 -> cfblk7/5(cfblk7)
  cfblk17/1 -> cfblk6/3(cfblk7)

== system sampleModel20/cfblk86/cfblk9/cfblk4 ==
  cfblk1 : Inport
  cfblk13 : Inport  Port=2
  cfblk14 : Inport  Port=3
  cfblk10 : Subsystem
  cfblk11 : Subsystem
  cfblk12 : Subsystem
  cfblk{17..23} (7 alike) : Delay  SampleTime=1
  cfblk3 : Polyval  Coefs=[ +2.081618890e-019, -1.441693666e-014, +4.719686976e-010, -8.536869453e-006, +1.621573104e-001, -8.087801117e+001 ]
  cfblk4 : Abs
  cfblk5 : Sum  Inputs=+-
  cfblk6 : Assignment  DiagnosticForDimensions=Warning  IndexOptions=Index vector (dialog)  Indices=1  OutputSizes=1
  cfblk7 : Math  Operator=hermitian  SaturateOnIntegerOverflow=on
  cfblk8 : Math  Operator=rem  SaturateOnIntegerOverflow=on
  cfblk9 : Subsystem
  cfblk2 : Outport
  cfblk15 : Outport  Port=2
  cfblk16 : Outport  Port=3
  wires:
  cfblk4/1 -> cfblk3/1, cfblk22/1
  cfblk13/1 -> cfblk11/1(cfblk1), cfblk6/2, cfblk11/5(cfblk9)
  cfblk10/1(cfblk2) -> cfblk5/1
  cfblk3/1 -> cfblk16/1, cfblk11/4(cfblk8)
  cfblk11/1(cfblk2) -> cfblk5/2
  cfblk1/1 -> cfblk2/1, cfblk8/2
  cfblk8/1 -> cfblk9/2(cfblk9)
  cfblk6/1 -> cfblk10/1(cfblk1), cfblk23/1
  cfblk7/1 -> cfblk10/2(cfblk9), cfblk11/2(cfblk6)
  cfblk11/2(cfblk11) -> cfblk10/3(cfblk10), cfblk15/1, cfblk19/1, cfblk20/1, cfblk21/1
  cfblk14/1 -> cfblk7/1, cfblk11/6(cfblk10)
  cfblk12/1(cfblk2) -> cfblk4/1, cfblk6/1, cfblk11/3(cfblk7)
  cfblk9/2(cfblk12) -> cfblk12/1(cfblk1)
  cfblk9/1(cfblk2) -> cfblk17/1
  cfblk17/1 -> cfblk8/1
  cfblk5/1 -> cfblk18/1
  cfblk18/1 -> cfblk9/1(cfblk1)
  cfblk19/1 -> cfblk9/3(cfblk10)
  cfblk20/1 -> cfblk12/2(cfblk9)
  cfblk21/1 -> cfblk12/4(cfblk11)
  cfblk22/1 -> cfblk9/4(cfblk11)
  cfblk23/1 -> cfblk12/3(cfblk10)

== system sampleModel20/cfblk86/cfblk9/cfblk5 ==
  cfblk1 : Inport
  cfblk13 : Inport  Port=2
  cfblk14 : Inport  Port=3
  cfblk15 : Inport  Port=4
  cfblk10 : Reshape
  cfblk11 : Subsystem
  cfblk12 : Subsystem
  cfblk16 : Delay  SampleTime=1
  cfblk17 : Delay  SampleTime=1
  cfblk3 : Product  Inputs=*
  cfblk4 : simulink/Math Operations/MinMax Running Resettable  Function=min  vinit=0.0
  cfblk5 : PermuteDimensions
  cfblk6 : Sum  Inputs=+-
  cfblk7 : Sin  TimeSource=Use external signal  SampleTime=0
  cfblk8 : Abs
  cfblk9 : Sqrt  Operator=rSqrt  AlgorithmType=Newton-Raphson  SaturateOnIntegerOverflow=on
  cfblk2 : Outport
  wires:
  cfblk11/1(cfblk2) -> cfblk2/1
  cfblk5/1 -> cfblk4/1
  cfblk3/1 -> cfblk8/1
  cfblk1/1 -> cfblk6/1, cfblk11/8(cfblk12)
  cfblk8/1 -> cfblk5/1, cfblk11/7(cfblk11)
  cfblk12/2(cfblk8) -> cfblk9/1
  cfblk7/1 -> cfblk4/2
  cfblk15/1 -> cfblk7/1
  cfblk6/1 -> cfblk3/1, cfblk11/6(cfblk10)
  cfblk10/1 -> cfblk6/2
  cfblk4/1 -> cfblk11/3(cfblk7), cfblk12/4(cfblk7)
  cfblk13/1 -> cfblk10/1, cfblk11/5(cfblk9)
  cfblk11/2(cfblk13) -> cfblk12/1(cfblk1)
  cfblk11/3(cfblk14) -> cfblk12/2(cfblk5)
  cfblk14/1 -> cfblk11/4(cfblk8)
  cfblk11/4(cfblk15) -> cfblk12/3(cfblk6)
  cfblk12/1(cfblk2) -> cfblk16/1
  cfblk16/1 -> cfblk11/1(cfblk1)
  cfblk9/1 -> cfblk17/1
  cfblk17/1 -> cfblk11/2(cfblk6)

== system sampleModel20/cfblk86/cfblk9/cfblk6 ==
  cfblk1 : Inport
  cfblk9 : Inport  Port=2
  cfblk{10..17} (8 alike) : Delay  SampleTime=1
  cfblk3 : Sum  Inputs=|++
  cfblk4 : Sum  Inputs=+
  cfblk5 : Abs
  cfblk6 : Subsystem
  cfblk7 : Subsystem
  cfblk8 : Subsystem
  cfblk2 : Outport
  wires:
  cfblk8/1(cfblk2) -> cfblk2/1
  cfblk8/2(cfblk12) -> cfblk3/1
  cfblk4/1 -> cfblk5/1, cfblk13/1, cfblk14/1, cfblk15/1
  cfblk7/1(cfblk2) -> cfblk6/1(cfblk1)
  cfblk3/1 -> cfblk7/1(cfblk1), cfblk17/1
  cfblk6/1(cfblk2) -> cfblk4/1, cfblk10/1
  cfblk8/3(cfblk13) -> cfblk7/2(cfblk11), cfblk6/3(cfblk9), cfblk7/5(cfblk14), cfblk7/6(cfblk15)
  cfblk9/1 -> cfblk8/1(cfblk1), cfblk6/2(cfblk8), cfblk8/5(cfblk10)
  cfblk1/1 -> cfblk8/2(cfblk7)
  cfblk5/1 -> cfblk11/1, cfblk12/1
  cfblk10/1 -> cfblk3/2
  cfblk11/1 -> cfblk7/3(cfblk12)
  cfblk12/1 -> cfblk8/6(cfblk11)
  cfblk13/1 -> cfblk6/4(cfblk10)
  cfblk14/1 -> cfblk7/4(cfblk13)
  cfblk15/1 -> cfblk6/5(cfblk11)
  cfblk7/2(cfblk16) -> cfblk16/1
  cfblk16/1 -> cfblk8/3(cfblk8)
  cfblk17/1 -> cfblk8/4(cfblk9)

== system sampleModel20/cfblk86/cfblk9/cfblk7 ==
  cfblk1 : Inport
  cfblk9 : Inport  Port=2
  cfblk10 : Delay  SampleTime=1
  cfblk11 : Delay  SampleTime=1
  cfblk3 : Product  Inputs=**
  cfblk4 : Sum  Inputs=|++
  cfblk5 : Sqrt  SaturateOnIntegerOverflow=on
  cfblk6 : DotProduct  InputSameDT=on  OutDataTypeStr=Inherit: Inherit via internal rule
  cfblk7 : UnaryMinus
  cfblk8 : Subsystem
  cfblk2 : Outport
  wires:
  cfblk9/1 -> cfblk7/1, cfblk8/3(cfblk12)
  cfblk1/1 -> cfblk4/1, cfblk8/4(cfblk13)
  cfblk7/1 -> cfblk8/1(cfblk1), cfblk6/2
  cfblk6/1 -> cfblk5/1, cfblk2/1, cfblk11/1
  cfblk4/1 -> cfblk8/2(cfblk11)
  cfblk8/1(cfblk2) -> cfblk6/1
  cfblk5/1 -> cfblk3/1
  cfblk8/2(cfblk15) -> cfblk3/2
  cfblk3/1 -> cfblk10/1
  cfblk10/1 -> cfblk4/2
  cfblk11/1 -> cfblk8/5(cfblk14)

== system sampleModel20/cfblk86/cfblk9/cfblk8 ==
  cfblk1 : Inport
  cfblk8 : Inport  Port=2
  cfblk9 : Inport  Port=3
  cfblk10 : Inport  Port=4
  cfblk11 : Inport  Port=5
  cfblk12 : Inport  Port=6
  cfblk13 : Inport  Port=7
  cfblk14 : Inport  Port=8
  cfblk15 : Delay  SampleTime=1
  cfblk16 : Delay  SampleTime=1
  cfblk17 : Delay  SampleTime=1
  cfblk3 : Product  Inputs=*
  cfblk4 : Subsystem
  cfblk5 : Subsystem
  cfblk6 : Subsystem
  cfblk7 : Subsystem
  cfblk2 : Outport
  wires:
  cfblk11/1 -> cfblk7/1(cfblk1)
  cfblk12/1 -> cfblk4/1(cfblk1), cfblk2/1, cfblk4/3(cfblk7)
  cfblk7/1(cfblk2) -> cfblk3/1
  cfblk9/1 -> cfblk7/2(cfblk11), cfblk4/5(cfblk9)
  cfblk5/1(cfblk2) -> cfblk6/2(cfblk7)
  cfblk6/1(cfblk2) -> cfblk4/4(cfblk8), cfblk15/1
  cfblk3/1 -> cfblk5/2(cfblk9), cfblk4/7(cfblk11)
  cfblk8/1 -> cfblk6/3(cfblk8), cfblk7/6(cfblk15), cfblk5/6(cfblk13), cfblk4/6(cfblk10)
  cfblk1/1 -> cfblk7/3(cfblk12)
  cfblk10/1 -> cfblk5/3(cfblk10)
  cfblk13/1 -> cfblk5/4(cfblk11)
  cfblk5/3(cfblk15) -> cfblk6/4(cfblk9)
  cfblk7/2(cfblk16) -> cfblk4/2(cfblk6)
  cfblk14/1 -> cfblk7/5(cfblk14)
  cfblk7/3(cfblk17) -> cfblk5/5(cfblk12)
  cfblk15/1 -> cfblk5/1(cfblk1)
  cfblk4/1(cfblk2) -> cfblk16/1
  cfblk16/1 -> cfblk6/1(cfblk1)
  cfblk5/2(cfblk14) -> cfblk17/1
  cfblk17/1 -> cfblk7/4(cfblk13)

== system sampleModel20/cfblk86/cfblk9/cfblk9 ==
  cfblk1 : Inport
  cfblk11 : Inport  Port=2
  cfblk12 : Inport  Port=3
  cfblk13 : Inport  Port=4
  cfblk10 : Subsystem
  cfblk{16..22} (7 alike) : Delay  SampleTime=1
  cfblk3 : PermuteDimensions
  cfblk4 : Trigonometry
  cfblk5 : Abs
  cfblk6 : Subsystem
  cfblk7 : Subsystem
  cfblk8 : Subsystem
  cfblk9 : Subsystem
  cfblk2 : Outport
  cfblk14 : Outport  Port=2
  cfblk15 : Outport  Port=3
  wires:
  cfblk5/1 -> cfblk2/1
  cfblk13/1 -> cfblk10/1(cfblk1)
  cfblk4/1 -> cfblk5/1
  cfblk7/1(cfblk2) -> cfblk3/1
  cfblk1/1 -> cfblk7/1(cfblk1), cfblk8/2(cfblk9)
  cfblk11/1 -> cfblk15/1
  cfblk8/2(cfblk11) -> cfblk14/1, cfblk19/1
  cfblk3/1 -> cfblk10/3(cfblk11), cfblk22/1
  cfblk7/2(cfblk13) -> cfblk8/1(cfblk1)
  cfblk10/1(cfblk2) -> cfblk6/1(cfblk1)
  cfblk6/2(cfblk14) -> cfblk4/1
  cfblk12/1 -> cfblk6/2(cfblk11), cfblk6/4(cfblk13)
  cfblk10/2(cfblk12) -> cfblk6/3(cfblk12)
  cfblk6/3(cfblk15) -> cfblk8/3(cfblk10), cfblk17/1
  cfblk10/3(cfblk13) -> cfblk9/1(cfblk1)
  cfblk10/4(cfblk14) -> cfblk9/2(cfblk7)
  cfblk10/5(cfblk15) -> cfblk9/3(cfblk8), cfblk21/1
  cfblk6/1(cfblk2) -> cfblk16/1
  cfblk16/1 -> cfblk7/3(cfblk8)
  cfblk17/1 -> cfblk7/4(cfblk9)
  cfblk8/1(cfblk2) -> cfblk18/1
  cfblk18/1 -> cfblk10/2(cfblk10)
  cfblk19/1 -> cfblk7/5(cfblk10)
  cfblk9/1(cfblk2) -> cfblk20/1
  cfblk20/1 -> cfblk7/2(cfblk7)
  cfblk21/1 -> cfblk7/7(cfblk12)
  cfblk22/1 -> cfblk7/6(cfblk11)

== system sampleModel20/cfblk87/cfblk5/cfblk10 ==
  cfblk1 : Inport
  cfblk7 : Inport  Port=2
  cfblk8 : Inport  Port=3
  cfblk9 : Inport  Port=4
  cfblk3 : Sqrt  Operator=rSqrt  AlgorithmType=Newton-Raphson  SaturateOnIntegerOverflow=on
  cfblk4 : DotProduct  InputSameDT=on  OutDataTypeStr=Inherit: Inherit via internal rule
  cfblk5 : Product  Inputs=*
  cfblk6 : Subsystem
  cfblk2 : Outport
  wires:
  cfblk9/1 -> cfblk3/1
  cfblk4/1 -> cfblk2/1
  cfblk8/1 -> cfblk5/1, cfblk6/3(cfblk11)
  cfblk3/1 -> cfblk4/1
  cfblk5/1 -> cfblk4/2
  cfblk1/1 -> cfblk6/1(cfblk1), cfblk6/4(cfblk12)
  cfblk7/1 -> cfblk6/2(cfblk10), cfblk6/5(cfblk13), cfblk6/6(cfblk14)

== system sampleModel20/cfblk87/cfblk5/cfblk11 ==
  cfblk1 : Inport
  cfblk11 : Inport  Port=2
  cfblk12 : Inport  Port=3
  cfblk13 : Inport  Port=4
  cfblk14 : Inport  Port=5
  cfblk15 : Inport  Port=6
  cfblk16 : Inport  Port=7
  cfblk10 : Subsystem
  cfblk{17..20} (4 alike) : Delay  SampleTime=1
  cfblk3 : simulink/Discrete/Transfer Fcn Real Zero  ZeroZ=0.75  ICPrevInput=0.0  DoSatur=off
      settings: SourceProductBaseCode=SL
  cfblk4 : Product  Inputs=*
  cfblk5 : Squeeze
  cfblk6 : MinMax  Function=max  Inputs=3
  cfblk7 : Trigonometry
  cfblk8 : Subsystem
  cfblk9 : Subsystem
  cfblk2 : Outport
  wires:
  cfblk3/1 -> cfblk5/1, cfblk10/5(cfblk14), cfblk8/3(cfblk8)
  cfblk13/1 -> cfblk4/1, cfblk8/5(cfblk10), cfblk8/8(cfblk13)
  cfblk11/1 -> cfblk10/1(cfblk1)
  cfblk7/1 -> cfblk2/1
  cfblk4/1 -> cfblk9/1(cfblk1)
  cfblk8/1(cfblk2) -> cfblk7/1
  cfblk15/1 -> cfblk9/2(cfblk11)
  cfblk14/1 -> cfblk6/1, cfblk8/4(cfblk9)
  cfblk12/1 -> cfblk3/1
  cfblk1/1 -> cfblk6/3, cfblk8/6(cfblk11)
  cfblk16/1 -> cfblk9/3(cfblk12)
  cfblk9/2(cfblk15) -> cfblk8/1(cfblk1)
  cfblk6/1 -> cfblk9/5(cfblk14)
  cfblk8/3(cfblk15) -> cfblk10/2(cfblk11)
  cfblk8/4(cfblk16) -> cfblk10/3(cfblk12)
  cfblk5/1 -> cfblk10/4(cfblk13)
  cfblk10/1(cfblk2) -> cfblk19/1, cfblk20/1
  cfblk9/1(cfblk2) -> cfblk17/1
  cfblk17/1 -> cfblk6/2
  cfblk8/2(cfblk14) -> cfblk18/1
  cfblk18/1 -> cfblk9/4(cfblk13)
  cfblk19/1 -> cfblk8/2(cfblk7)
  cfblk20/1 -> cfblk8/7(cfblk12)

== system sampleModel20/cfblk87/cfblk5/cfblk7 ==
  cfblk1 : Inport
  cfblk8 : Inport  Port=2
  cfblk9 : Inport  Port=3
  cfblk10 : Inport  Port=4
  cfblk11 : Inport  Port=5
  cfblk12 : Inport  Port=6
  cfblk13 : Inport  Port=7
  cfblk15 : Delay  SampleTime=1
  cfblk3 : Sum  Inputs=--
  cfblk4 : Bias  Bias=[-616961338.805001]
  cfblk5 : PermuteDimensions
  cfblk6 : simulink/Math Operations/MinMax Running Resettable  Function=min  vinit=0.0
  cfblk7 : Subsystem
  cfblk2 : Outport
  cfblk14 : Outport  Port=2
  wires:
  cfblk6/1 -> cfblk4/1
  cfblk10/1 -> cfblk3/2
  cfblk11/1 -> cfblk7/1(cfblk1)
  cfblk1/1 -> cfblk7/2(cfblk4), cfblk7/5(cfblk7)
  cfblk13/1 -> cfblk7/3(cfblk5)
  cfblk12/1 -> cfblk14/1
  cfblk4/1 -> cfblk5/1
  cfblk3/1 -> cfblk6/1
  cfblk8/1 -> cfblk6/2, cfblk7/7(cfblk9)
  cfblk9/1 -> cfblk7/4(cfblk6), cfblk7/6(cfblk8)
  cfblk7/1(cfblk2) -> cfblk2/1
  cfblk5/1 -> cfblk15/1
  cfblk15/1 -> cfblk3/1

== system sampleModel20/cfblk87/cfblk5/cfblk8 ==
  cfblk1 : Inport
  cfblk11 : Inport  Port=2
  cfblk12 : Inport  Port=3
  cfblk13 : Inport  Port=4
  cfblk14 : Inport  Port=5
  cfblk10 : Subsystem
  cfblk{16..19} (4 alike) : Delay  SampleTime=1
  cfblk3 : pid_lib/PID Controller (2DOF)  Controller=PID  Form=Parallel  TimeDomain=Discrete-time  UseExternalTs=off  SampleTime=1  IntegratorMethod=Forward Euler  FilterMethod=Forward Euler  ControllerParametersSource=internal  P=1  I=1  D=0  UseFilter=on  N=100  b=1  c=1  TunerSelectOption=Transfer Function Based (PID Tuner App)  InitialConditionSource=internal  InitialConditionForIntegrator=0  InitialConditionForFilter=0  DifferentiatorICPrevScaledInput=0  ExternalReset=none  TrackingMode=off  Kt=1  LimitOutput=off  SatLimitsSource=internal  UpperSaturationLimit=inf  LowerSaturationLimit=-inf  LinearizeAsGain=off  AntiWindupMode=none  Kb=1  POutMin=[]  POutMax=[]  IOutMin=[]  IOutMax=[]  DOutMin=[]  DOutMax=[]  NOutMin=[]  NOutMax=[]  bOutMin=[]  bOutMax=[]  cOutMin=[]  cOutMax=[]  SumOutMin=[]  SumOutMax=[]  SaturationOutMin=[]  SaturationOutMax=[]  PParamMin=[]  PParamMax=[]  IParamMin=[]  IParamMax=[]  DParamMin=[]  DParamMax=[]  NParamMin=[]  NParamMax=[]  bParamMin=[]  bParamMax=[]  cParamMin=[]  cParamMax=[]  KbParamMin=[]  KbParamMax=[]  KtParamMin=[]  KtParamMax=[]  KbOutMin=[]  KbOutMax=[]  KtOutMin=[]  KtOutMax=[]  IntegratorOutMin=[]  IntegratorOutMax=[]  FilterOutMin=[]  FilterOutMax=[]  SumI1OutMin=[]  SumI1OutMax=[]  SumI2OutMin=[]  SumI2OutMax=[]  SumI3OutMin=[]  SumI3OutMax=[]  SumI4OutMin=[]  SumI4OutMax=[]  SumDOutMin=[]  SumDOutMax=[]  Sum1OutMin=[]  Sum1OutMax=[]  Sum2OutMin=[]  Sum2OutMax=[]  Sum3OutMin=[]  Sum3OutMax=[]  DifferentiatorOutMin=[]  DifferentiatorOutMax=[]  FilterDiffOutCoefMin=[]  FilterDiffOutCoefMax=[]  ReciprocalOutMin=[]  ReciprocalOutMax=[]  SumDenOutMin=[]  SumDenOutMax=[]  SumNumOutMin=[]  SumNumOutMax=[]  DivideOutMin=[]  DivideOutMax=[]  UdiffTsProdOutMin=[]  UdiffTsProdOutMax=[]  NTsProdOutMin=[]  NTsProdOutMax=[]  UintegralTsProdOutMin=[]  UintegralTsProdOutMax=[]  UngainTsProdOutMin=[]  UngainTsProdOutMax=[]  IntegratorContinuousStateAttributes=''  IntegratorStateMustResolveToSignalObject=off  IntegratorRTWStateStorageClass=Auto  FilterContinuousStateAttributes=''  FilterStateMustResolveToSignalObject=off  FilterRTWStateStorageClass=Auto  ParallelPVariant=InternalParameters  IdealPVariant=Disabled  IVariant=InternalParameters  DVariant=InternalParameters  bVariant=InternalParameters  cVariant=InternalParameters  IntegratorVariant=Discrete  SatVariant=Disabled  AWVariant=Passthrough  PCopyVariant=Disabled  TRVariant=Disabled  FdbkBlocksVariant=Forward  IdealPFdbkVariant=Disabled  SatFdbkVariant=Disabled  DerivativeFilterVariant=ForwardEulerFilter  NVariant=InternalParameters  NCopyVariant=Disabled  FilterICVariant=InternalICsFilter  IntegratorICVariant=InternalICs  ExternalResetVariant=Disabled  TRSumVariant=Passthrough  SumFdbkVariant=Disabled  SumVariant=Sum_PID  TsampFilterVariant=InternalTs  TsampNgainVariant=Passthrough  TsampIntegralVariant=Passthrough  ExternalSaturationOutDataTypeStr=Inherit: Same as second input
      settings: SourceProductBaseCode=SL
  cfblk4 : ComplexToRealImag
  cfblk5 : UnaryMinus
  cfblk6 : UnaryMinus
  cfblk7 : Subsystem
  cfblk8 : Subsystem
  cfblk9 : Subsystem
  cfblk2 : Outport
  cfblk15 : Outport  Port=2
  wires:
  cfblk5/1 -> cfblk2/1
  cfblk7/1(cfblk2) -> cfblk10/1(cfblk1), cfblk17/1
  cfblk12/1 -> cfblk7/1(cfblk1)
  cfblk13/1 -> cfblk5/1
  cfblk4/1 -> cfblk10/2(cfblk9)
  cfblk11/1 -> cfblk7/2(cfblk10)
  cfblk9/1(cfblk2) -> cfblk6/1
  cfblk8/1(cfblk2) -> cfblk9/1(cfblk1)
  cfblk14/1 -> cfblk3/1
  cfblk3/1 -> cfblk15/1
  cfblk1/1 -> cfblk8/1(cfblk1)
  cfblk9/2(cfblk10) -> cfblk7/3(cfblk11)
  cfblk10/1(cfblk2) -> cfblk3/2
  cfblk9/3(cfblk11) -> cfblk4/1
  cfblk8/2(cfblk10) -> cfblk7/4(cfblk12)
  cfblk8/3(cfblk11) -> cfblk9/3(cfblk8), cfblk9/4(cfblk9)
  cfblk9/4(cfblk12) -> cfblk7/5(cfblk13), cfblk19/1
  cfblk6/1 -> cfblk16/1
  cfblk16/1 -> cfblk9/2(cfblk7)
  cfblk17/1 -> cfblk8/4(cfblk9)
  cfblk4/2 -> cfblk18/1
  cfblk18/1 -> cfblk8/2(cfblk7)
  cfblk19/1 -> cfblk8/3(cfblk8)

== system sampleModel20/cfblk87/cfblk5/cfblk9 ==
  cfblk1 : Inport
  cfblk7 : Inport  Port=2
  cfblk8 : Inport  Port=3
  cfblk9 : Inport  Port=4
  cfblk10 : Inport  Port=5
  cfblk11 : Inport  Port=6
  cfblk12 : Inport  Port=7
  cfblk13 : Inport  Port=8
  cfblk14 : Inport  Port=9
  cfblk15 : Inport  Port=10
  cfblk17 : Delay  SampleTime=1
  cfblk3 : Reshape
  cfblk4 : Sqrt  SaturateOnIntegerOverflow=on
  cfblk5 : Subsystem
  cfblk6 : Subsystem
  cfblk2 : Outport
  cfblk16 : Outport  Port=2
  wires:
  cfblk13/1 -> cfblk6/1(cfblk1), cfblk5/8(cfblk13)
  cfblk8/1 -> cfblk6/2(cfblk7)
  cfblk1/1 -> cfblk3/1
  cfblk9/1 -> cfblk16/1, cfblk5/9(cfblk14)
  cfblk11/1 -> cfblk5/1(cfblk1)
  cfblk15/1 -> cfblk4/1
  cfblk14/1 -> cfblk6/3(cfblk8), cfblk5/7(cfblk12)
  cfblk5/1(cfblk2) -> cfblk6/4(cfblk9)
  cfblk12/1 -> cfblk2/1
  cfblk10/1 -> cfblk5/2(cfblk7)
  cfblk3/1 -> cfblk5/4(cfblk9)
  cfblk7/1 -> cfblk5/5(cfblk10), cfblk5/10(cfblk15)
  cfblk4/1 -> cfblk5/6(cfblk11)
  cfblk6/1(cfblk2) -> cfblk17/1
  cfblk17/1 -> cfblk5/3(cfblk8)

== system sampleModel20/cfblk87/cfblk6/cfblk10 ==
  cfblk1 : Inport
  cfblk8 : Inport  Port=2
  cfblk9 : Inport  Port=3
  cfblk10 : Inport  Port=4
  cfblk11 : Inport  Port=5
  cfblk{13..18} (6 alike) : Delay  SampleTime=1
  cfblk3 : Sqrt  Operator=rSqrt  AlgorithmType=Newton-Raphson  SaturateOnIntegerOverflow=on
  cfblk4 : Subsystem
  cfblk5 : Subsystem
  cfblk6 : Subsystem
  cfblk7 : Subsystem
  cfblk2 : Outport
  cfblk12 : Outport  Port=2
  wires:
  cfblk9/1 -> cfblk4/1(cfblk1), cfblk5/5(cfblk10)
  cfblk8/1 -> cfblk12/1, cfblk4/4(cfblk10)
  cfblk5/1(cfblk2) -> cfblk3/1
  cfblk7/1(cfblk2) -> cfblk4/2(cfblk8)
  cfblk1/1 -> cfblk7/1(cfblk1), cfblk6/3(cfblk6)
  cfblk11/1 -> cfblk5/1(cfblk1)
  cfblk4/1(cfblk2) -> cfblk6/1(cfblk1)
  cfblk10/1 -> cfblk4/3(cfblk9), cfblk7/4(cfblk8)
  cfblk4/2(cfblk11) -> cfblk2/1
  cfblk6/1(cfblk2) -> cfblk5/3(cfblk8)
  cfblk4/3(cfblk12) -> cfblk5/4(cfblk9)
  cfblk5/3(cfblk12) -> cfblk15/1, cfblk16/1
  cfblk6/2(cfblk7) -> cfblk17/1, cfblk18/1
  cfblk3/1 -> cfblk13/1
  cfblk13/1 -> cfblk5/2(cfblk7)
  cfblk5/2(cfblk11) -> cfblk14/1
  cfblk14/1 -> cfblk7/2(cfblk6)
  cfblk15/1 -> cfblk6/2(cfblk5)
  cfblk16/1 -> cfblk7/5(cfblk9)
  cfblk17/1 -> cfblk7/3(cfblk7)
  cfblk18/1 -> cfblk7/6(cfblk10)

== system sampleModel20/cfblk87/cfblk6/cfblk11 ==
  cfblk1 : Inport
  cfblk6 : Inport  Port=2
  cfblk7 : Inport  Port=3
  cfblk8 : Inport  Port=4
  cfblk9 : Inport  Port=5
  cfblk10 : Inport  Port=6
  cfblk14 : Delay  SampleTime=1
  cfblk15 : Delay  SampleTime=1
  cfblk16 : Delay  SampleTime=1
  cfblk3 : Sum  Inputs=+-
  cfblk4 : Subsystem
  cfblk5 : Subsystem
  cfblk2 : Outport
  cfblk11 : Outport  Port=2
  cfblk12 : Outport  Port=3
  cfblk13 : Outport  Port=4
  wires:
  cfblk1/1 -> cfblk4/1(cfblk1)
  cfblk10/1 -> cfblk11/1
  cfblk8/1 -> cfblk4/2(cfblk6)
  cfblk4/1(cfblk2) -> cfblk2/1
  cfblk4/2(cfblk9) -> cfblk3/1
  cfblk7/1 -> cfblk5/1(cfblk1)
  cfblk4/3(cfblk10) -> cfblk5/2(cfblk9)
  cfblk6/1 -> cfblk5/3(cfblk10)
  cfblk4/4(cfblk11) -> cfblk5/4(cfblk11), cfblk5/6(cfblk13), cfblk5/7(cfblk14)
  cfblk3/1 -> cfblk5/5(cfblk12)
  cfblk9/1 -> cfblk12/1
  cfblk5/2(cfblk15) -> cfblk13/1
  cfblk5/3(cfblk16) -> cfblk15/1, cfblk16/1
  cfblk5/1(cfblk2) -> cfblk14/1
  cfblk14/1 -> cfblk4/3(cfblk7)
  cfblk15/1 -> cfblk4/4(cfblk8)
  cfblk16/1 -> cfblk3/2

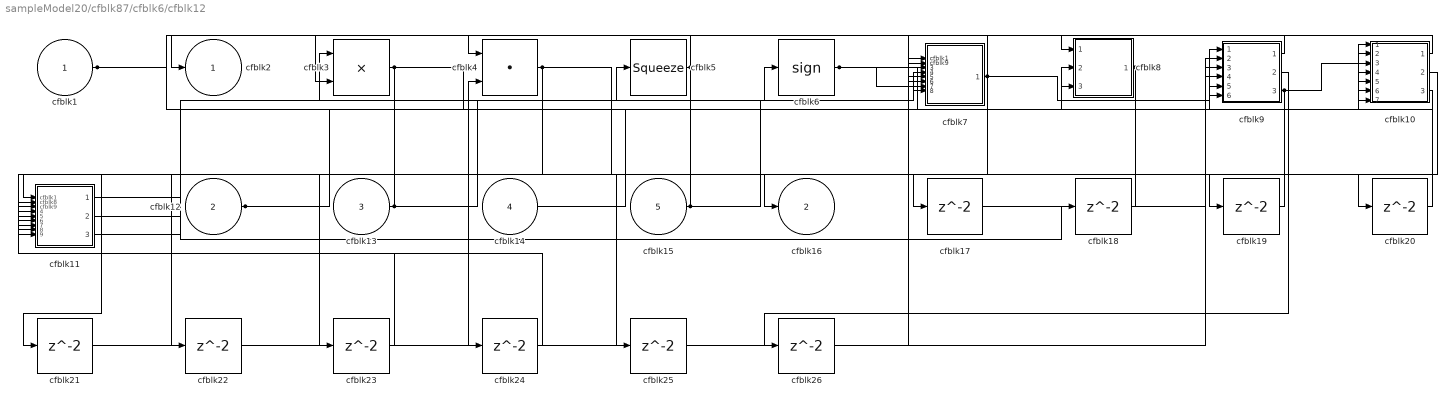
== system sampleModel20/cfblk87/cfblk6/cfblk12 ==
  cfblk1 : Inport
  cfblk12 : Inport  Port=2
  cfblk13 : Inport  Port=3
  cfblk14 : Inport  Port=4
  cfblk15 : Inport  Port=5
  cfblk10 : Subsystem
  cfblk11 : Subsystem
  cfblk{17..26} (10 alike) : Delay  SampleTime=1
  cfblk3 : Product
  cfblk4 : DotProduct  InputSameDT=on  OutDataTypeStr=Inherit: Inherit via internal rule
  cfblk5 : Squeeze
  cfblk6 : Signum
  cfblk7 : Subsystem
  cfblk8 : Subsystem
  cfblk9 : Subsystem
  cfblk2 : Outport
  cfblk16 : Outport  Port=2
  wires:
  cfblk3/1 -> cfblk11/1(cfblk1), cfblk10/5(cfblk7)
  cfblk13/1 -> cfblk6/1, cfblk11/3(cfblk9)
  cfblk10/1(cfblk2) -> cfblk8/1(cfblk1)
  cfblk7/1(cfblk2) -> cfblk2/1, cfblk9/5(cfblk12), cfblk11/4(cfblk10), cfblk11/7(cfblk13), cfblk11/9(cfblk15)
  cfblk10/2(cfblk10) -> cfblk16/1
  cfblk6/1 -> cfblk10/1(cfblk1), cfblk7/7(cfblk14)
  cfblk14/1 -> cfblk9/1(cfblk1)
  cfblk10/3(cfblk11) -> cfblk8/2(cfblk7)
  cfblk15/1 -> cfblk3/1, cfblk11/2(cfblk8), cfblk7/4(cfblk11), cfblk7/8(cfblk15), cfblk11/5(cfblk11)
  cfblk9/1(cfblk2) -> cfblk3/2
  cfblk4/1 -> cfblk10/6(cfblk8), cfblk19/1, cfblk20/1, cfblk21/1
  cfblk9/3(cfblk15) -> cfblk8/3(cfblk8), cfblk10/3(cfblk5)
  cfblk5/1 -> cfblk4/1, cfblk25/1
  cfblk11/3(cfblk17) -> cfblk5/1
  cfblk12/1 -> cfblk10/2(cfblk4), cfblk9/6(cfblk13), cfblk10/4(cfblk6)
  cfblk1/1 -> cfblk7/3(cfblk10), cfblk10/7(cfblk9)
  cfblk8/1(cfblk2) -> cfblk22/1, cfblk23/1, cfblk24/1
  cfblk11/1(cfblk2) -> cfblk17/1
  cfblk17/1 -> cfblk9/3(cfblk10)
  cfblk11/2(cfblk16) -> cfblk18/1
  cfblk18/1 -> cfblk7/2(cfblk9)
  cfblk19/1 -> cfblk9/2(cfblk9)
  cfblk20/1 -> cfblk7/5(cfblk12)
  cfblk21/1 -> cfblk7/6(cfblk13)
  cfblk22/1 -> cfblk4/2
  cfblk23/1 -> cfblk11/6(cfblk12)
  cfblk24/1 -> cfblk11/8(cfblk14)
  cfblk25/1 -> cfblk9/4(cfblk11)
  cfblk9/2(cfblk14) -> cfblk26/1
  cfblk26/1 -> cfblk7/1(cfblk1)
